simulink model "observer_model"  (R2024a)
settings: Solver=FixedStepAuto  StartTime=0.0  StopTime=3  FixedStep=0.0001  RelTol=1e-3
values from neighbouring files (symbols this model uses):
  A = [5 -5 -9 3; -5 5 -3 9; -9 -3 5 5; 3 9 5 5]    [ex.m]    (also in observer.m = [20 5 -16 9; 6 1 -4 1; 32 9 -25 14; 8 4 -6 4]; observer_down.m; reg.m = [2 3; -3 2])
  C = [1 -1 1 1; 1 3 -1 3]    [ex.m]    (also in observer.m = [-1 0 1 -1]; observer_down.m = [0 0 0 1; 0 1 0 0])
  L1 = inv(Q1)*Y1    [observer.m]
  L3 = inv(Q3)*Y3    [observer.m]
settings Model: Creator=ventus  LastModifiedBy=ventus
settings OptimizationCC: EnhancedBackFolding=on  PassReuseOutputArgsAs=Individual arguments  ZeroExternalMemoryAtStartup=off  ZeroInternalMemoryAtStartup=off  MaxStackSize=64  OptimizeBlockOrder=speed  DifferentSizesBufferReuse=on  OptimizationCustomize=off  EfficientTunableParamExpr=on
settings DebuggingCC: ParameterTunabilityLossMsg=error
settings SFSimCC: MATLABDynamicMemAlloc=off
settings RTWCC: Description=Embedded Coder  SystemTargetFile=ert.tlc  HardwareBoard=Robot Operating System 2 (ROS 2)  TLCOptions="-aInlineSetEventsForThisBaseRateFcn=TLC_FALSE -aSuppressMultiTaskScheduler=TLC_FALSE  -aRateBasedStepFcn=0"  TemplateMakefile=ert_default_tmf  Toolchain=Colcon Tools  TargetLang=C++
settings CodeAppCC: ForceParamTrailComments=on  IgnoreCustomStorageClasses=off  OperatorAnnotations=on  SimulinkDataObjDesc=on  SFDataObjDesc=on  InsertBlockDesc=on
settings ERTTargetCC: CodeInterfacePackaging=C++ class  RootIOFormat=Structure reference

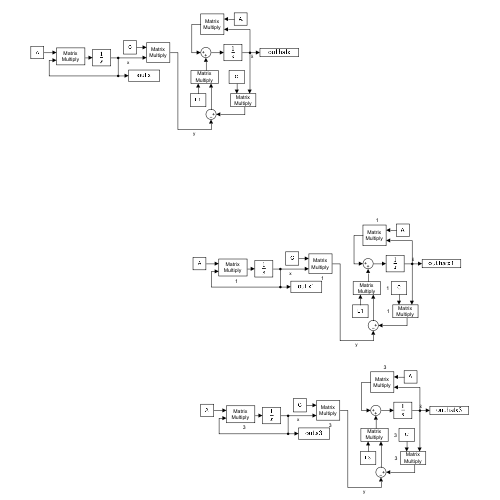
[thumbnail: Simulink's stored preview of the top-level diagram]
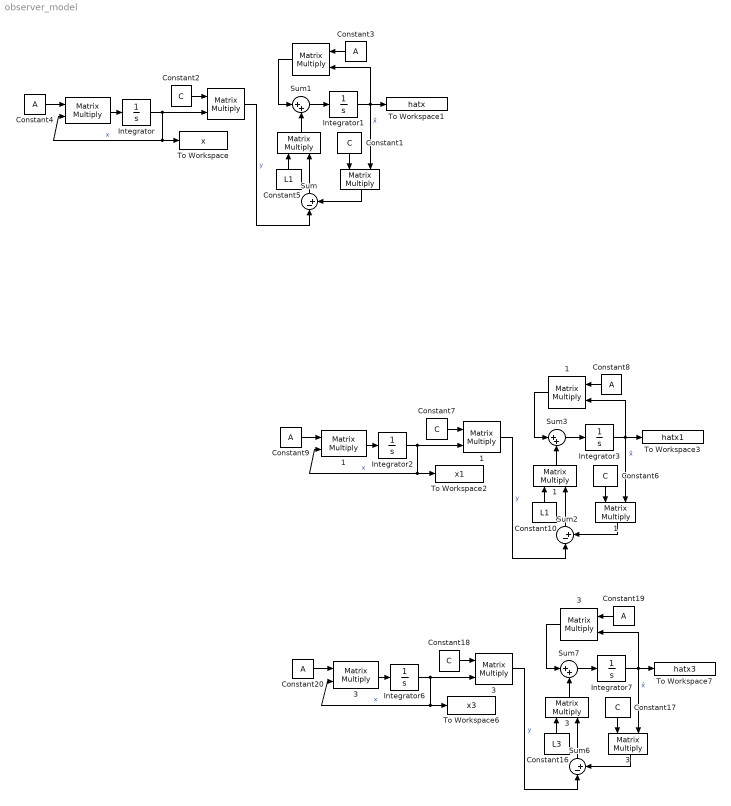
== system observer_model ==
  " " : Product  Multiplication=Matrix(*)
  "  " : Product  Multiplication=Matrix(*)
  "   " : Product  Multiplication=Matrix(*)
  "    " : Product  Multiplication=Matrix(*)
  "     " : Product  Multiplication=Matrix(*)
  "     1" : Product  Multiplication=Matrix(*)
  "     3" : Product  Multiplication=Matrix(*)
  "    1" : Product  Multiplication=Matrix(*)
  "    3" : Product  Multiplication=Matrix(*)
  "   1" : Product  Multiplication=Matrix(*)
  "   3" : Product  Multiplication=Matrix(*)
  "  1" : Product  Multiplication=Matrix(*)
  "  3" : Product  Multiplication=Matrix(*)
  " 1" : Product  Multiplication=Matrix(*)
  " 3" : Product  Multiplication=Matrix(*)
  Constant{1..2,6..7,17..18} (6 alike) : Constant  Value=C  VectorParams1D=off
  Constant10 : Constant  Value=L1  VectorParams1D=off
  Constant16 : Constant  Value=L3  VectorParams1D=off
  Constant{3..4,8..9,19..20} (6 alike) : Constant  Value=A  VectorParams1D=off
  Constant5 : Constant  Value=L1  VectorParams1D=off
  Integrator : Integrator  InitialCondition=[1; 1; 1; 1]
  Integrator1 : Integrator  InitialCondition=[2; 0; 0; -1]
  Integrator2 : Integrator  InitialCondition=[1; 1; 1; 1]
  Integrator3 : Integrator  InitialCondition=[2; 0; 0; -1]
  Integrator6 : Integrator  InitialCondition=[1; 1; 1; 1]
  Integrator7 : Integrator  InitialCondition=[2; 0; 0; -1]
  Sum : Sum  Inputs=|-+
  Sum1 : Sum  Inputs=|++
  Sum2 : Sum  Inputs=|-+
  Sum3 : Sum  Inputs=|++
  Sum6 : Sum  Inputs=|-+
  Sum7 : Sum  Inputs=|++
  To Workspace : ToWorkspace  VariableName=x  SaveFormat=Timeseries  SampleTime=-1
  To Workspace1 : ToWorkspace  VariableName=hatx  SaveFormat=Timeseries  SampleTime=-1
  To Workspace2 : ToWorkspace  VariableName=x1  SaveFormat=Timeseries  SampleTime=-1
  To Workspace3 : ToWorkspace  VariableName=hatx1  SaveFormat=Timeseries  SampleTime=-1
  To Workspace6 : ToWorkspace  VariableName=x3  SaveFormat=Timeseries  SampleTime=-1
  To Workspace7 : ToWorkspace  VariableName=hatx3  SaveFormat=Timeseries  SampleTime=-1
  wires:
  Integrator/1 -> "   "/2, To Workspace/1, "     "/2  "x"
  Integrator1/1 -> To Workspace1/1, "    "/2, " "/2  "x̂"
  "   "/1 -> Sum/1  "y"
  "    "/1 -> Sum1/1
  Sum1/1 -> Integrator1/1
  "     "/1 -> Integrator/1
  " "/1 -> Sum/2
  Constant5/1 -> "  "/1
  Sum/1 -> "  "/2
  "  "/1 -> Sum1/2
  Constant3/1 -> "    "/1
  Constant4/1 -> "     "/1
  Constant2/1 -> "   "/1
  Constant1/1 -> " "/1
  Integrator2/1 -> "   1"/2, To Workspace2/1, "     1"/2  "x"
  Constant8/1 -> "    1"/1
  Sum2/1 -> "  1"/2
  " 1"/1 -> Sum2/2
  Constant10/1 -> "  1"/1
  Sum3/1 -> Integrator3/1
  Constant7/1 -> "   1"/1
  "     1"/1 -> Integrator2/1
  "  1"/1 -> Sum3/2
  Constant9/1 -> "     1"/1
  "   1"/1 -> Sum2/1  "y"
  "    1"/1 -> Sum3/1
  Constant6/1 -> " 1"/1
  Integrator3/1 -> To Workspace3/1, "    1"/2, " 1"/2  "x̂"
  Integrator7/1 -> To Workspace7/1, "    3"/2, " 3"/2  "x̂"
  Constant17/1 -> " 3"/1
  Sum7/1 -> Integrator7/1
  " 3"/1 -> Sum6/2
  Constant19/1 -> "    3"/1
  Integrator6/1 -> "   3"/2, To Workspace6/1, "     3"/2  "x"
  "    3"/1 -> Sum7/1
  "   3"/1 -> Sum6/1  "y"
  Constant20/1 -> "     3"/1
  Sum6/1 -> "  3"/2
  "  3"/1 -> Sum7/2
  "     3"/1 -> Integrator6/1
  Constant18/1 -> "   3"/1
  Constant16/1 -> "  3"/1
